simulink model "furutaobs"  (Simulink 9.1)
settings: Solver=ode5  StartTime=0.0  StopTime=10.0  FixedStep=.005  MaxStep=0.01  RelTol=1e-3  EnableMultiTasking=on
values from neighbouring files (symbols this model uses):
  Ad = DiscSYS.A    [PolePlace.m]
  Bd = DiscSYS.B    [PolePlace.m]
  Cd = DiscSYS.C    [PolePlace.m]
  Kd = [-8.5445,-3.3264,-94.3109,-12.4099]    [PolePlace.m]
  L = place(DiscSYS.A',DiscSYS.C',ozp)'    [PolePlace.m]
settings Model: Creator=ayush2  LastModifiedBy=ayush2
settings DataIOCC: LimitDataPoints=on  SignalLoggingSaveFormat=ModelDataLogs  SignalLoggingName=sigsOut
settings OptimizationCC: LifeSpan=auto
settings DebuggingCC: SaveWithParameterizedLinksMsg=none  SignalResolutionControl=TryResolveAllWithWarning  MultiTaskDSMMsg=warning  MultiTaskCondExecSysMsg=none  SFUnexpectedBacktrackingDiag=error  SFNoUnconditionalDefaultTransitionDiag=error  SFExecutionAtInitializationDiag=warning
settings HardwareCC: TargetUnknown=on
settings CodeAppCC: StateflowObjectComments=off

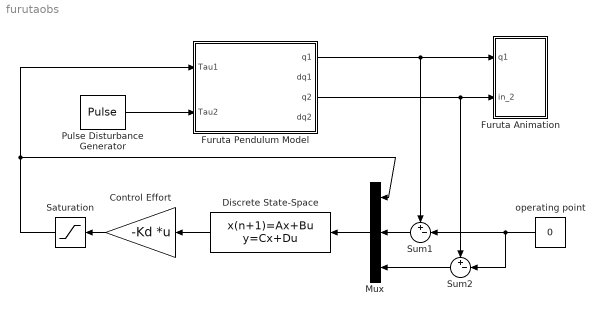
== system furutaobs ==
  Control Effort : Gain  Gain=-Kd  Multiplication=Matrix(K*u)  SaturateOnIntegerOverflow=on  OutDataTypeStr=Inherit: Same as input  ParamDataTypeStr=Inherit: Same as input
  Discrete State-Space : DiscreteStateSpace  A=[Ad-L*Cd]  B=[Bd L]  C=eye(4)  D=zeros(4,3)  SampleTime=.005
  Furuta Animation : Subsystem
  Furuta Pendulum Model : Subsystem  mask{par=[0.0363 0.0306 0.0356 0.0260 0.3829], g=9.804, init=[0 0 0 0]}
      mask prompts: par "parameters"; g "acceleration of gravity"; init "Initial Conditions"
  Mux : Mux  Inputs=3
  Pulse Disturbance Generator : DiscretePulseGenerator  PulseType=Time based  Amplitude=1.5  Period=4  PulseWidth=4  PhaseDelay=4
  Saturation : Saturate  UpperLimit=10  LowerLimit=-10
  Sum1 : Sum  Inputs=+-|  SaturateOnIntegerOverflow=on
  Sum2 : Sum  Inputs=+-|  SaturateOnIntegerOverflow=on
  operating point : Constant  Value=0
  wires:
  Furuta Pendulum Model/1(q1) -> Furuta Animation/1(q1), Sum1/1
  Furuta Pendulum Model/3(q2) -> Sum2/1, Furuta Animation/2(in_2)
  Pulse Disturbance Generator/1 -> Furuta Pendulum Model/2(Tau2)
  Control Effort/1 -> Saturation/1
  Discrete State-Space/1 -> Control Effort/1
  Mux/1 -> Discrete State-Space/1
  Sum1/1 -> Mux/2
  Sum2/1 -> Mux/3
  operating point/1 -> Sum1/2, Sum2/2
  Saturation/1 -> Mux/1, Furuta Pendulum Model/1(Tau1)

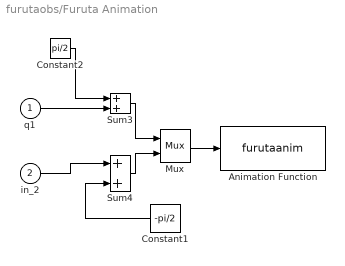
== system furutaobs/Furuta Animation ==
  q1 : Inport
  in_2 : Inport  Port=2
  Animation Function : S-Function  FunctionName=furutaanim  Parameters=0.05  SFunctionDeploymentMode=off  EnableBusSupport=off
      settings: DeleteFcn=if ~isempty(findobj('type','figure','name','dblpend1 Animation'));close('dblpend1 Animation'); end;
  Constant1 : Constant  Value=-pi/2
  Constant2 : Constant  Value=pi/2
  Mux : Mux  Inputs=2
  Sum3 : Sum  SaturateOnIntegerOverflow=on  InputSameDT=on  OutDataTypeStr=Inherit: Same as first input
  Sum4 : Sum  SaturateOnIntegerOverflow=on  InputSameDT=on  OutDataTypeStr=Inherit: Same as first input
  wires:
  q1/1 -> Sum3/2
  Constant2/1 -> Sum3/1
  Sum3/1 -> Mux/1
  Sum4/1 -> Mux/2
  Mux/1 -> Animation Function/1
  Constant1/1 -> Sum4/2
  in_2/1 -> Sum4/1

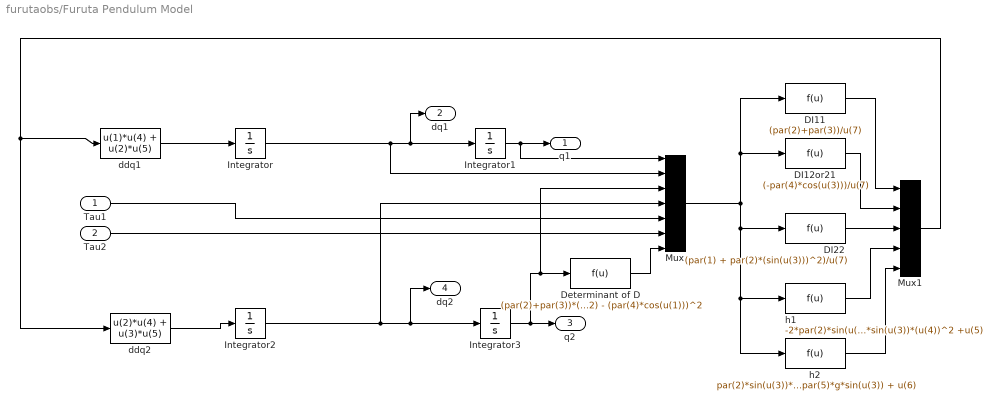
== system furutaobs/Furuta Pendulum Model ==
  Tau1 : Inport
  Tau2 : Inport  Port=2
  DI11 : Fcn  Expr=(par(2)+par(3))/u(7)
  DI12or21 : Fcn  Expr=(-par(4)*cos(u(3)))/u(7)
  DI22 : Fcn  Expr=(par(1) + par(2)*(sin(u(3)))^2)/u(7)
  Determinant of D : Fcn  Expr=(par(2)+par(3))*(par(1) + par(2)*(sin(u(1)))^2) - (par(4)*cos(u(1)))^2
  Integrator : Integrator  InitialCondition=init(2)
  Integrator1 : Integrator  InitialCondition=init(1)
  Integrator2 : Integrator  InitialCondition=init(4)
  Integrator3 : Integrator  InitialCondition=init(3)
  Mux : Mux  Inputs=7
  Mux1 : Mux  Inputs=5
  ddq1 : Fcn  Expr=u(1)*u(4) + u(2)*u(5)
  ddq2 : Fcn  Expr=u(2)*u(4) + u(3)*u(5)
  h1 : Fcn  Expr=-2*par(2)*sin(u(3))*cos(u(3))*u(2)*u(4)+par(4)*sin(u(3))*(u(4))^2 +u(5)
  h2 : Fcn  Expr=par(2)*sin(u(3))*cos(u(3))*(u(2))^2 + par(5)*g*sin(u(3)) + u(6)
  q1 : Outport
  dq1 : Outport  Port=2
  q2 : Outport  Port=3
  dq2 : Outport  Port=4
  wires:
  Determinant of D/1 -> Mux/7
  ddq1/1 -> Integrator/1
  ddq2/1 -> Integrator2/1
  Mux1/1 -> ddq1/1, ddq2/1
  DI11/1 -> Mux1/1
  DI12or21/1 -> Mux1/2
  h2/1 -> Mux1/5
  h1/1 -> Mux1/4
  DI22/1 -> Mux1/3
  Mux/1 -> DI12or21/1, DI11/1, DI22/1, h1/1, h2/1
  Tau1/1 -> Mux/5
  Tau2/1 -> Mux/6
  Integrator2/1 -> Mux/4, dq2/1, Integrator3/1
  Integrator/1 -> Mux/2, dq1/1, Integrator1/1
  Integrator1/1 -> Mux/1, q1/1
  Integrator3/1 -> Mux/3, Determinant of D/1, q2/1
